simulink model "SC_ChgModel"  (R2022b)
settings: Solver=VariableStepAuto  StartTime=0.0  StopTime=inf  RelTol=1e-3
undefined symbols (not defined in the file or in its folder): sc_charge_limit, sc_discharge_limit, sc_E, SC_iv, SC_nm, SC_np, SC_ns, SC_rc, SC_SocTable
settings Model: Creator=xuupp  LastModifiedBy=xuupp
settings DataIOCC: SaveFormat=Array  SaveOutput=off  SignalLogging=off  DSMLogging=off  SaveTime=off  ReturnWorkspaceOutputs=off

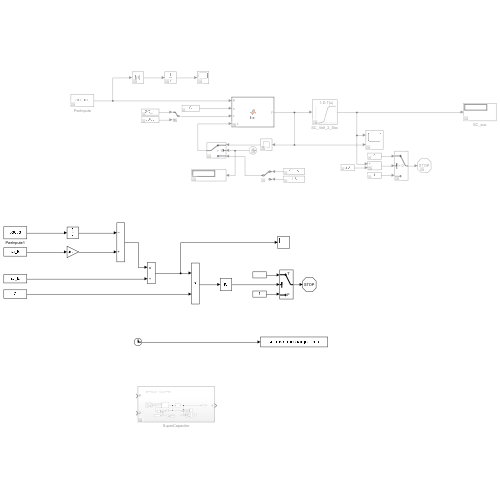
[thumbnail: Simulink's stored preview of the top-level diagram]
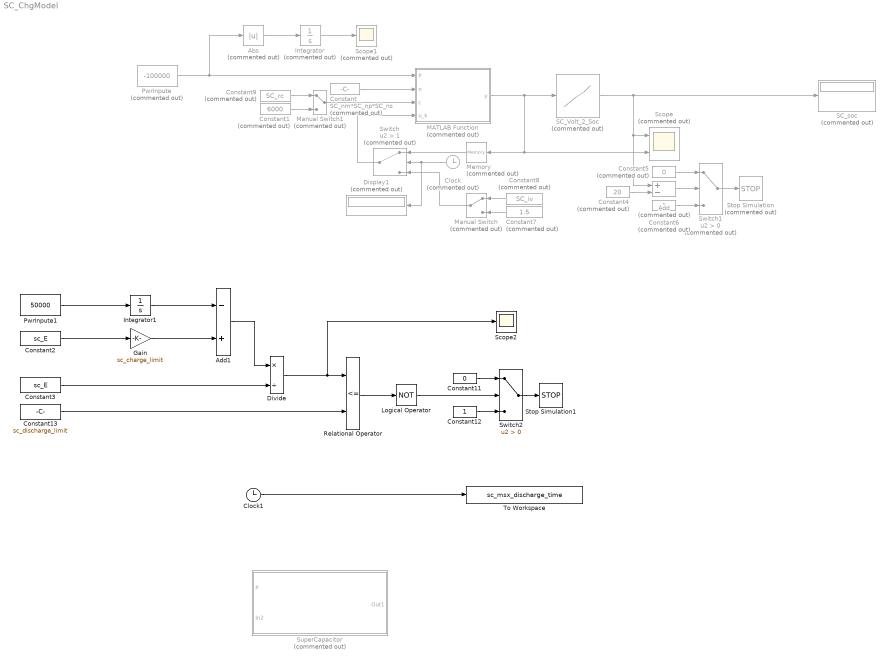
== system SC_ChgModel ==
  Abs : Abs  Commented=on  SaturateOnIntegerOverflow=off
  Add : Sum  Commented=on  Inputs=+-
  Add1 : Sum  Inputs=-+
  Clock : Clock  Commented=on
  Clock1 : Clock
  Constant : Constant  Commented=on  Value=SC_nm*SC_np*SC_ns
  Constant1 : Constant  Commented=on  Value=6000
  Constant11 : Constant  Value=0
  Constant12 : Constant
  Constant13 : Constant  Value=sc_discharge_limit
  Constant2 : Constant  Value=sc_E
  Constant3 : Constant  Value=sc_E
  Constant4 : Constant  Commented=on  Value=20
  Constant5 : Constant  Commented=on  Value=0
  Constant6 : Constant  Commented=on
  Constant7 : Constant  Commented=on  Value=1.5
  Constant8 : Constant  Commented=on  Value=SC_iv
  Constant9 : Constant  Commented=on  Value=SC_rc
  Display1 : Display  Commented=on
  Divide : Product  Inputs=*/
  Gain : Gain  Gain=sc_charge_limit
  Integrator : Integrator  Commented=on
  Integrator1 : Integrator
  Logical Operator : Logic  Operator=NOT  AllPortsSameDT=off  OutDataTypeStr=boolean
  MATLAB Function : MATLAB Function  Commented=on  TreatAsAtomicUnit=on
  Manual Switch : ManualSwitch  Commented=on
  Manual Switch1 : ManualSwitch  Commented=on
  Memory : Memory  Commented=on
  PwrInpute : Constant  Commented=on  Value=-100000
  PwrInpute1 : Constant  Value=50000
  Relational Operator : RelationalOperator  Operator=<=  OutDataTypeStr=boolean  RndMeth=Simplest  InputSameDT=off
  SC_Volt_2_Soc : Lookup_n-D  Commented=on  NumberOfTableDimensions=1  BreakpointsForDimension1=SC_SocTable(:,1)  Table=SC_SocTable(:,2)  InternalRulePriority=Speed  RndMeth=Simplest
  SC_soc : Display  Commented=on
  Scope : Scope  Commented=on  NumInputPorts=2
  Scope1 : Scope  Commented=on
  Scope2 : Scope
  Stop Simulation : Stop  Commented=on
  Stop Simulation1 : Stop
  SuperCapacitor : Subsystem  Commented=on
  Switch : Switch  Commented=on  Criteria=u2 > Threshold  Threshold=1  SaturateOnIntegerOverflow=off  InputSameDT=off
  Switch1 : Switch  Commented=on  Criteria=u2 > Threshold  SaturateOnIntegerOverflow=off  InputSameDT=off
  Switch2 : Switch  Criteria=u2 > Threshold  SaturateOnIntegerOverflow=off  InputSameDT=off
  To Workspace : ToWorkspace  VariableName=sc_msx_discharge_time  SampleTime=-1
      settings: Save2DSignal=2-D array (concatenate along first dimension)
  wires:
  MATLAB Function/1(y) -> Memory/1, Scope/2, SC_Volt_2_Soc/1
  SC_Volt_2_Soc/1 -> SC_soc/1, Add/1, Scope/1
  Memory/1 -> Switch/1
  Manual Switch/1 -> Switch/3
  Clock/1 -> Display1/1, Switch/2
  Switch/1 -> MATLAB Function/4(u_k)
  Constant/1 -> MATLAB Function/2(n)
  Manual Switch1/1 -> MATLAB Function/3(c)
  PwrInpute/1 -> Abs/1, MATLAB Function/1(P)
  Switch1/1 -> Stop Simulation/1
  Add/1 -> Switch1/2
  Constant4/1 -> Add/2
  Constant5/1 -> Switch1/1
  Constant6/1 -> Switch1/3
  Constant7/1 -> Manual Switch/2
  Constant8/1 -> Manual Switch/1
  Constant9/1 -> Manual Switch1/1
  Constant1/1 -> Manual Switch1/2
  Abs/1 -> Integrator/1
  Integrator/1 -> Scope1/1
  PwrInpute1/1 -> Integrator1/1
  Integrator1/1 -> Add1/1
  Constant2/1 -> Gain/1
  Add1/1 -> Divide/1
  Clock1/1 -> To Workspace/1
  Constant3/1 -> Divide/2
  Constant12/1 -> Switch2/3
  Constant11/1 -> Switch2/1
  Logical Operator/1 -> Switch2/2
  Switch2/1 -> Stop Simulation1/1
  Divide/1 -> Scope2/1, Relational Operator/1
  Gain/1 -> Add1/2
  Constant13/1 -> Relational Operator/2
  Relational Operator/1 -> Logical Operator/1

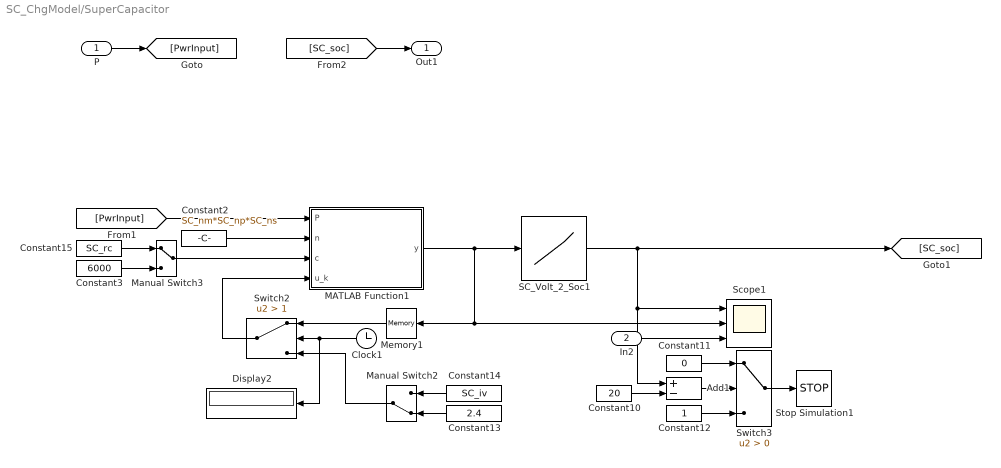
== system SC_ChgModel/SuperCapacitor ==
  P : Inport
  In2 : Inport  Port=2
  Add1 : Sum  Inputs=+-
  Clock1 : Clock
  Constant10 : Constant  Value=20
  Constant11 : Constant  Value=0
  Constant12 : Constant
  Constant13 : Constant  Value=2.4
  Constant14 : Constant  Value=SC_iv
  Constant15 : Constant  Value=SC_rc
  Constant2 : Constant  Value=SC_nm*SC_np*SC_ns
  Constant3 : Constant  Value=6000
  Display2 : Display
  MATLAB Function1 : MATLAB Function  TreatAsAtomicUnit=on
  Manual Switch2 : ManualSwitch  CurrentSetting=0
  Manual Switch3 : ManualSwitch
  Memory1 : Memory
  SC_Volt_2_Soc1 : Lookup_n-D  NumberOfTableDimensions=1  BreakpointsForDimension1=SC_SocTable(:,1)  Table=SC_SocTable(:,2)  InternalRulePriority=Speed  RndMeth=Simplest
  Scope1 : Scope  NumInputPorts=3
  Stop Simulation1 : Stop
  Switch2 : Switch  Criteria=u2 > Threshold  Threshold=1  SaturateOnIntegerOverflow=off  InputSameDT=off
  Switch3 : Switch  Criteria=u2 > Threshold  SaturateOnIntegerOverflow=off  InputSameDT=off
  Out1 : Outport
  wires:
  Switch3/1 -> Stop Simulation1/1
  Constant12/1 -> Switch3/3
  Constant10/1 -> Add1/2
  SC_Volt_2_Soc1/1 -> [SC_soc], Scope1/1, Add1/1
  Constant3/1 -> Manual Switch3/2
  P/1 -> [PwrInput]
  Clock1/1 -> Switch2/2, Display2/1
  MATLAB Function1/1(y) -> SC_Volt_2_Soc1/1, Scope1/2, Memory1/1
  Add1/1 -> Switch3/2
  Constant15/1 -> Manual Switch3/1
  Constant14/1 -> Manual Switch2/1
  Constant11/1 -> Switch3/1
  Constant2/1 -> MATLAB Function1/2(n)
  Manual Switch2/1 -> Switch2/3
  Constant13/1 -> Manual Switch2/2
  Memory1/1 -> Switch2/1
  Switch2/1 -> MATLAB Function1/4(u_k)
  Manual Switch3/1 -> MATLAB Function1/3(c)
  In2/1 -> Scope1/3
  [PwrInput] -> MATLAB Function1/1(P)
  [SC_soc] -> Out1/1

== matlab function SC_ChgModel/SuperCapacitor/MATLAB Function1 ==
  data: P input; y output; n input; c input; u_k input
function y = fcn(P,n,c,u_k)

y = (2*P/(n*c)+(u_k)^2)^(1/2);

== matlab function SC_ChgModel/MATLAB Function ==
  data: P input; y output; n input; c input; u_k input
function y = fcn(P,n,c,u_k)

y = (2*P/(n*c)+(u_k)^2)^(1/2);
